simulink model "L4T1_FullWaveBridgeRectifier_follows_Reference"  (R2021a)
settings: Solver=VariableStepAuto  StartTime=0.0  StopTime=2  RelTol=1e-3  EnableMultiTasking=on
libraries: spsThyristorLib x4, spsVoltageMeasurementLib x2, spsACVoltageSourceLib x1, spsMeanLib x1, spsPLLLib x1, spsSampleandHoldLib x1, spsSeriesRLCBranchLib x1, spspowerguiLib x1
settings Model: Creator=COMLAB-18  LastModifiedBy=hp
settings SolverCC: AlgebraicLoopSolver=TrustRegion
settings DataIOCC: ReturnWorkspaceOutputs=off
settings OptimizationCC: LifeSpan=inf
settings DebuggingCC: SFUnexpectedBacktrackingDiag=warning  SFNoUnconditionalDefaultTransitionDiag=warning  SFMachineParentedDataDiag=warning  ArithmeticOperatorsInVariantConditions=warning
settings SFSimCC: SimUseLocalCustomCode=off  CustomCodeUndefinedFunction=UseInterfaceOnly
settings RTWCC: RTWUseLocalCustomCode=off
settings CodeAppCC: StateflowObjectComments=on
settings GRTTargetCC: TargetLangStandard=C89/C90 (ANSI)
settings ConfigComp: CovMetricSettings=dw  CovSaveCumulativeToWorkspaceVar=on  CovSaveSingleToWorkspaceVar=on  CovExternalEMLEnable=off
settings SimscapeCC: SimscapeNormalizeSystem=off

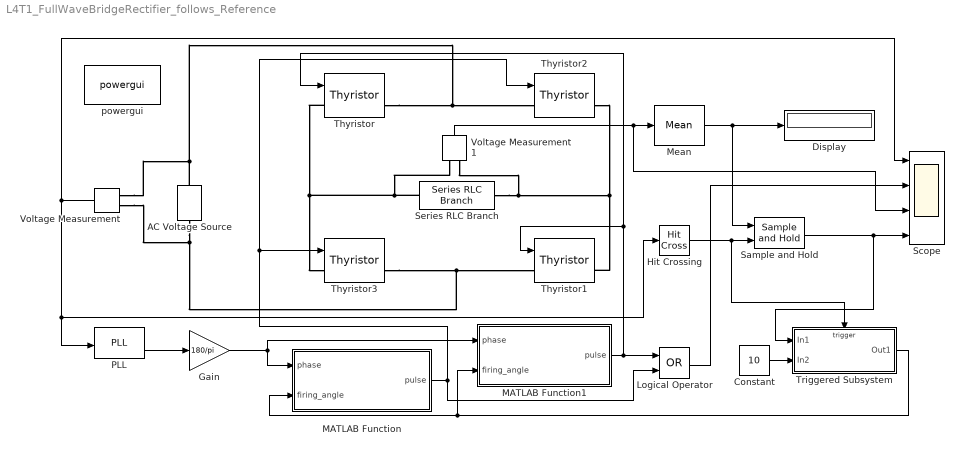
== system L4T1_FullWaveBridgeRectifier_follows_Reference ==
  AC Voltage Source : spsACVoltageSourceLib/AC Voltage Source  Amplitude=100  Phase=0  Frequency=50  SampleTime=0  Measurements=None  BusType=swing  Pref=10e3  Qref=0  Qmin=-inf  Qmax=+inf
  Constant : Constant  Value=10
  Display : Display
  Gain : Gain  Gain=180/pi
  Hit Crossing : HitCross  HitCrossingDirection=rising
  Logical Operator : Logic  Operator=OR  AllPortsSameDT=off  OutDataTypeStr=boolean
  MATLAB Function : MATLAB Function  TreatAsAtomicUnit=on
  MATLAB Function1 : MATLAB Function  TreatAsAtomicUnit=on
  Mean : spsMeanLib/Mean  Freq=50  Vinit=0  Ts=0
  PLL : spsPLLLib/PLL  Fmin=45  Par_Init=[0, 50]  ParK=[180, 3200, 1]  TcD=1e-4  MaxRateChangeFreq=12  FilterCutOffFreq=25  Ts=0  AGC=on
      settings: SourceProductBaseCode=PS
  Sample and Hold : spsSampleandHoldLib/Sample and Hold  ic=0  Ts=0
      settings: SourceProductBaseCode=PS
  Scope : Scope  NumInputPorts=4
  Series RLC Branch : spsSeriesRLCBranchLib/Series RLC Branch  LConnTagsString=__new0  RConnTagsString=__new0  BranchType=R  Resistance=10  Inductance=1e-3  SetiL0=off  InitialCurrent=0  Capacitance=1e-6  Setx0=off  InitialVoltage=0  Measurements=None
  Thyristor{,1..3} (4 alike) : spsThyristorLib/Thyristor  Ron=0.001  Lon=0  Vf=0.8  IC=0  Rs=500  Cs=250e-9  Measurements=on
  Triggered Subsystem : Subsystem  TreatAsAtomicUnit=on
  Voltage Measurement : spsVoltageMeasurementLib/Voltage Measurement  PhasorSimulation=off  OutputType=Complex  PSBequivalent=0
  Voltage Measurement1 : spsVoltageMeasurementLib/Voltage Measurement  PhasorSimulation=off  OutputType=Complex  PSBequivalent=0
  powergui : spspowerguiLib/powergui  Priority=1  SimulationMode=Discrete  SampleTime=50e-6  frequency=60  Iterations=50  frequencyindice=50  Pbase=100e6  ErrMax=1e-4  UnitsV=kV  UnitsW=MW  buscounter=0  FunctionMessages=off  echomessages=off  EnableUseOfTLC=off  CurrentSourceSwitches=off  DisableSnubberDevices=off  DisableRonSwitches=off  DisableVfSwitches=off  DisplayEquations=off  AutomaticDiscreteSolvers=off  SolverType=Tustin/Backward Euler (TBE)  Interpol=off  ExternalGateDelay=off  methode=off  Ts=10  x0status=blocks  SPID=off  SwTol=0  HookPort=off  NonlinearTolerance=1e-4  nMaxIteration=100  ContinueOnMaxIteration=off  RestoreLinks=warning  ResistiveCurrentMeasurement=off  Frange=[0:2:500]  Ylog=off  Xlog=on  ShowGrid=off  save=off  variable=ZData  structure=0  ZoomFFT=off  StartTime=0.0  cycles=1  DisplayStyle=1  fundamental=60  FreqAxis=off  MaxFrequency=1000  frequencyindicesteady=1  RmsSteady=1  display=off
  wires:
  Voltage Measurement/1 -> Hit Crossing/1, PLL/1, Scope/1
  PLL/2 -> Gain/1
  Mean/1 -> Sample and Hold/1, Display/1
  Hit Crossing/1 -> Triggered Subsystem/Trigger, Sample and Hold/2
  Gain/1 -> MATLAB Function1/1(phase), MATLAB Function/1(phase)
  Constant/1 -> Triggered Subsystem/2(In2)
  Sample and Hold/1 -> Triggered Subsystem/1(In1), Scope/4
  Triggered Subsystem/1(Out1) -> MATLAB Function1/2(firing_angle), MATLAB Function/2(firing_angle)
  MATLAB Function/1(pulse) -> Logical Operator/2, Thyristor3/1, Thyristor2/1
  MATLAB Function1/1(pulse) -> Thyristor/1, Thyristor1/1, Logical Operator/1
  Logical Operator/1 -> Scope/2
  Voltage Measurement1/1 -> Scope/3, Mean/1
  connections:
  Thyristor/RConn1 -- Voltage Measurement/LConn1 -- AC Voltage Source/RConn1 -- Thyristor2/LConn1
  Thyristor3/RConn1 -- AC Voltage Source/LConn1 -- Voltage Measurement/LConn2 -- Thyristor1/LConn1
  Thyristor/LConn1 -- Series RLC Branch/RConn1 -- Voltage Measurement1/LConn2 -- Thyristor3/LConn1
  Thyristor2/RConn1 -- Voltage Measurement1/LConn1 -- Series RLC Branch/LConn1 -- Thyristor1/RConn1

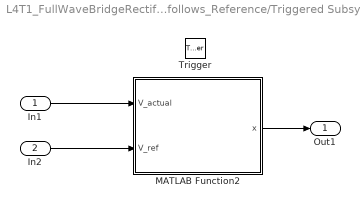
== system L4T1_FullWaveBridgeRectifier_follows_Reference/Triggered Subsystem ==
  In1 : Inport
  In2 : Inport  Port=2
  Trigger : TriggerPort  VariantControl=Variant
  MATLAB Function2 : MATLAB Function  TreatAsAtomicUnit=on
  Out1 : Outport
  wires:
  In1/1 -> MATLAB Function2/1(V_actual)
  MATLAB Function2/1(x) -> Out1/1
  In2/1 -> MATLAB Function2/2(V_ref)

== matlab function L4T1_FullWaveBridgeRectifier_follows_Reference/MATLAB Function ==
  data: phase input; pulse output; firing_angle input
function pulse = fcn(phase,firing_angle)
d=5;
if phase>=firing_angle && phase<=min(firing_angle+d,180)
    pulse=1;
else
    pulse=0;
end
end

== matlab function L4T1_FullWaveBridgeRectifier_follows_Reference/Triggered Subsystem/MATLAB Function2 ==
  data: V_actual input; x output; V_ref input
function x = fcn(V_actual,V_ref)
d=5;
persistent firing_angle;
if isempty (firing_angle)
    firing_angle=10;
end
if V_actual<V_ref
    firing_angle=firing_angle-d;
    if firing_angle<0
        firing_angle=0;
    end
elseif V_actual==V_ref
    firing_angle=firing_angle;
else
    firing_angle=firing_angle+d;
    if firing_angle>180
        firing_angle=180;
    end
end
x=firing_angle;
end

== matlab function L4T1_FullWaveBridgeRectifier_follows_Reference/MATLAB Function1 ==
  data: phase input; pulse output; firing_angle input
function pulse = fcn(phase,firing_angle)
d=5;
if phase>=firing_angle+180 && phase<=min(firing_angle+180+d,360)
    pulse=1;
else
    pulse=0;
end
end
